simulink model "openWaterModel"  (R2020a)
settings: Solver=FixedStepAuto  StartTime=0.0  StopTime=inf  FixedStep=Ts  RelTol=1e-3  EnableMultiTasking=on
values from neighbouring files (symbols this model uses):
  ctrlMap =     [init_Kite.mat]
  Ts = 0.01    [init_Kite.mat]
undefined symbols (not defined in the file or in its folder): initializeBussesFromBlock, IO397, standard
libraries: xpcutilitieslib x172, hdlsllib x100, simulink x36, dspsigops x13, slrtlib x4, xpcseriallib x3, speedgoatlib_fpga_analog_io x2, xpcrtudplib x2, speedgoatlib_fpga_dio x1, speedgoatlib_fpga_quadrature x1, speedgoatlib_IO581 x1, speedgoatlib_fpga x1
(part 4 of 4)

== system openWaterModel/Sensor Processing/IMU Processing/Kite Measurements /binary2double3 ==
  In1 : Inport
  In2 : Inport  Port=2
  In3 : Inport  Port=3
  In4 : Inport  Port=4
  Bit Packing {,1..4} (5 alike) : xpcutilitieslib/Bit Packing 
      settings: SourceProductBaseCode=XP
  Bit Shift1 : hdlsllib/Logic and Bit Operations/Bit Shift  mode=Shift Left Logical  N=16
  Bit Shift2 : hdlsllib/Logic and Bit Operations/Bit Shift  mode=Shift Left Logical  N=24
  Bit Shift3 : hdlsllib/Logic and Bit Operations/Bit Shift  mode=Shift Left Logical  N=8
  Bitwise Operator : simulink/Logic and Bit Operations/Bitwise Operator  logicop=OR  UseBitMask=off  NumInputPorts=4  BitMask=bin2dec('00000000')  BitMaskRealWorld=Stored Integer
  Cast To Double1 : DataTypeConversion  OutDataTypeStr=double
  Display{3,5..7,10..14} (9 alike) : Display
      settings: Format=hex (Stored Integer)
  Double : Outport
  wires:
  Bit Shift1/1 -> Bitwise Operator/2, Display10/1
  Bitwise Operator/1 -> Display14/1, "Bit Packing "/1
  Bit Packing 1/1 -> Bit Shift2/1
  Bit Packing 4/1 -> Bitwise Operator/4, Display13/1
  In1/1 -> Bit Packing 1/1, Display3/1
  In3/1 -> Bit Packing 3/1, Display6/1
  Bit Shift2/1 -> Bitwise Operator/1, Display11/1
  Bit Packing 2/1 -> Bit Shift1/1
  "Bit Packing "/1 -> Cast To Double1/1
  Bit Shift3/1 -> Bitwise Operator/3, Display12/1
  Bit Packing 3/1 -> Bit Shift3/1
  In2/1 -> Bit Packing 2/1, Display5/1
  In4/1 -> Bit Packing 4/1, Display7/1
  Cast To Double1/1 -> Double/1

== system openWaterModel/Sensor Processing/IMU Processing/Kite Measurements /binary2double4 ==
  In1 : Inport
  In2 : Inport  Port=2
  In3 : Inport  Port=3
  In4 : Inport  Port=4
  Bit Packing {,1..4} (5 alike) : xpcutilitieslib/Bit Packing 
      settings: SourceProductBaseCode=XP
  Bit Shift1 : hdlsllib/Logic and Bit Operations/Bit Shift  mode=Shift Left Logical  N=16
  Bit Shift2 : hdlsllib/Logic and Bit Operations/Bit Shift  mode=Shift Left Logical  N=24
  Bit Shift3 : hdlsllib/Logic and Bit Operations/Bit Shift  mode=Shift Left Logical  N=8
  Bitwise Operator : simulink/Logic and Bit Operations/Bitwise Operator  logicop=OR  UseBitMask=off  NumInputPorts=4  BitMask=bin2dec('00000000')  BitMaskRealWorld=Stored Integer
  Cast To Double1 : DataTypeConversion  OutDataTypeStr=double
  Display{3,5..7,10..14} (9 alike) : Display
      settings: Format=hex (Stored Integer)
  Double : Outport
  wires:
  Bit Shift1/1 -> Bitwise Operator/2, Display10/1
  Bitwise Operator/1 -> Display14/1, "Bit Packing "/1
  Bit Packing 1/1 -> Bit Shift2/1
  Bit Packing 4/1 -> Bitwise Operator/4, Display13/1
  In1/1 -> Bit Packing 1/1, Display3/1
  In3/1 -> Bit Packing 3/1, Display6/1
  Bit Shift2/1 -> Bitwise Operator/1, Display11/1
  Bit Packing 2/1 -> Bit Shift1/1
  "Bit Packing "/1 -> Cast To Double1/1
  Bit Shift3/1 -> Bitwise Operator/3, Display12/1
  Bit Packing 3/1 -> Bit Shift3/1
  In2/1 -> Bit Packing 2/1, Display5/1
  In4/1 -> Bit Packing 4/1, Display7/1
  Cast To Double1/1 -> Double/1

== system openWaterModel/Sensor Processing/IMU Processing/Kite Measurements /binary2double5 ==
  In1 : Inport
  In2 : Inport  Port=2
  In3 : Inport  Port=3
  In4 : Inport  Port=4
  Bit Packing {,1..4} (5 alike) : xpcutilitieslib/Bit Packing 
      settings: SourceProductBaseCode=XP
  Bit Shift1 : hdlsllib/Logic and Bit Operations/Bit Shift  mode=Shift Left Logical  N=16
  Bit Shift2 : hdlsllib/Logic and Bit Operations/Bit Shift  mode=Shift Left Logical  N=24
  Bit Shift3 : hdlsllib/Logic and Bit Operations/Bit Shift  mode=Shift Left Logical  N=8
  Bitwise Operator : simulink/Logic and Bit Operations/Bitwise Operator  logicop=OR  UseBitMask=off  NumInputPorts=4  BitMask=bin2dec('00000000')  BitMaskRealWorld=Stored Integer
  Cast To Double1 : DataTypeConversion  OutDataTypeStr=double
  Display{3,5..7,10..14} (9 alike) : Display
      settings: Format=hex (Stored Integer)
  Double : Outport
  wires:
  Bit Shift1/1 -> Bitwise Operator/2, Display10/1
  Bitwise Operator/1 -> Display14/1, "Bit Packing "/1
  Bit Packing 1/1 -> Bit Shift2/1
  Bit Packing 4/1 -> Bitwise Operator/4, Display13/1
  In1/1 -> Bit Packing 1/1, Display3/1
  In3/1 -> Bit Packing 3/1, Display6/1
  Bit Shift2/1 -> Bitwise Operator/1, Display11/1
  Bit Packing 2/1 -> Bit Shift1/1
  "Bit Packing "/1 -> Cast To Double1/1
  Bit Shift3/1 -> Bitwise Operator/3, Display12/1
  Bit Packing 3/1 -> Bit Shift3/1
  In2/1 -> Bit Packing 2/1, Display5/1
  In4/1 -> Bit Packing 4/1, Display7/1
  Cast To Double1/1 -> Double/1

== system openWaterModel/Sensor Processing/IMU Processing/Kite Measurements /binary2double6 ==
  In1 : Inport
  In2 : Inport  Port=2
  In3 : Inport  Port=3
  In4 : Inport  Port=4
  Bit Packing {,1..4} (5 alike) : xpcutilitieslib/Bit Packing 
      settings: SourceProductBaseCode=XP
  Bit Shift1 : hdlsllib/Logic and Bit Operations/Bit Shift  mode=Shift Left Logical  N=16
  Bit Shift2 : hdlsllib/Logic and Bit Operations/Bit Shift  mode=Shift Left Logical  N=24
  Bit Shift3 : hdlsllib/Logic and Bit Operations/Bit Shift  mode=Shift Left Logical  N=8
  Bitwise Operator : simulink/Logic and Bit Operations/Bitwise Operator  logicop=OR  UseBitMask=off  NumInputPorts=4  BitMask=bin2dec('00000000')  BitMaskRealWorld=Stored Integer
  Cast To Double1 : DataTypeConversion  OutDataTypeStr=double
  Display{3,5..7,10..14} (9 alike) : Display
      settings: Format=hex (Stored Integer)
  Double : Outport
  wires:
  Bit Shift1/1 -> Bitwise Operator/2, Display10/1
  Bitwise Operator/1 -> Display14/1, "Bit Packing "/1
  Bit Packing 1/1 -> Bit Shift2/1
  Bit Packing 4/1 -> Bitwise Operator/4, Display13/1
  In1/1 -> Bit Packing 1/1, Display3/1
  In3/1 -> Bit Packing 3/1, Display6/1
  Bit Shift2/1 -> Bitwise Operator/1, Display11/1
  Bit Packing 2/1 -> Bit Shift1/1
  "Bit Packing "/1 -> Cast To Double1/1
  Bit Shift3/1 -> Bitwise Operator/3, Display12/1
  Bit Packing 3/1 -> Bit Shift3/1
  In2/1 -> Bit Packing 2/1, Display5/1
  In4/1 -> Bit Packing 4/1, Display7/1
  Cast To Double1/1 -> Double/1

== system openWaterModel/Sensor Processing/IMU Processing/Kite Measurements /binary2double7 ==
  In1 : Inport
  In2 : Inport  Port=2
  In3 : Inport  Port=3
  In4 : Inport  Port=4
  Bit Packing {,1..4} (5 alike) : xpcutilitieslib/Bit Packing 
      settings: SourceProductBaseCode=XP
  Bit Shift1 : hdlsllib/Logic and Bit Operations/Bit Shift  mode=Shift Left Logical  N=16
  Bit Shift2 : hdlsllib/Logic and Bit Operations/Bit Shift  mode=Shift Left Logical  N=24
  Bit Shift3 : hdlsllib/Logic and Bit Operations/Bit Shift  mode=Shift Left Logical  N=8
  Bitwise Operator : simulink/Logic and Bit Operations/Bitwise Operator  logicop=OR  UseBitMask=off  NumInputPorts=4  BitMask=bin2dec('00000000')  BitMaskRealWorld=Stored Integer
  Cast To Double1 : DataTypeConversion  OutDataTypeStr=double
  Display{3,5..7,10..14} (9 alike) : Display
      settings: Format=hex (Stored Integer)
  Double : Outport
  wires:
  Cast To Double1/1 -> Double/1
  In4/1 -> Display7/1, Bit Packing 4/1
  In2/1 -> Display5/1, Bit Packing 2/1
  Bit Packing 3/1 -> Bit Shift3/1
  Bit Shift3/1 -> Display12/1, Bitwise Operator/3
  "Bit Packing "/1 -> Cast To Double1/1
  Bit Packing 2/1 -> Bit Shift1/1
  Bit Shift2/1 -> Display11/1, Bitwise Operator/1
  In3/1 -> Display6/1, Bit Packing 3/1
  In1/1 -> Display3/1, Bit Packing 1/1
  Bit Packing 4/1 -> Display13/1, Bitwise Operator/4
  Bit Packing 1/1 -> Bit Shift2/1
  Bitwise Operator/1 -> "Bit Packing "/1, Display14/1
  Bit Shift1/1 -> Display10/1, Bitwise Operator/2

== system openWaterModel/Sensor Processing/IMU Processing/Kite Measurements /binary2double8 ==
  In1 : Inport
  In2 : Inport  Port=2
  In3 : Inport  Port=3
  In4 : Inport  Port=4
  Bit Packing {,1..4} (5 alike) : xpcutilitieslib/Bit Packing 
      settings: SourceProductBaseCode=XP
  Bit Shift1 : hdlsllib/Logic and Bit Operations/Bit Shift  mode=Shift Left Logical  N=16
  Bit Shift2 : hdlsllib/Logic and Bit Operations/Bit Shift  mode=Shift Left Logical  N=24
  Bit Shift3 : hdlsllib/Logic and Bit Operations/Bit Shift  mode=Shift Left Logical  N=8
  Bitwise Operator : simulink/Logic and Bit Operations/Bitwise Operator  logicop=OR  UseBitMask=off  NumInputPorts=4  BitMask=bin2dec('00000000')  BitMaskRealWorld=Stored Integer
  Cast To Double1 : DataTypeConversion  OutDataTypeStr=double
  Display{3,5..7,10..14} (9 alike) : Display
      settings: Format=hex (Stored Integer)
  Double : Outport
  wires:
  Bit Shift1/1 -> Bitwise Operator/2, Display10/1
  Bitwise Operator/1 -> Display14/1, "Bit Packing "/1
  Bit Packing 1/1 -> Bit Shift2/1
  Bit Packing 4/1 -> Bitwise Operator/4, Display13/1
  In1/1 -> Bit Packing 1/1, Display3/1
  In3/1 -> Bit Packing 3/1, Display6/1
  Bit Shift2/1 -> Bitwise Operator/1, Display11/1
  Bit Packing 2/1 -> Bit Shift1/1
  "Bit Packing "/1 -> Cast To Double1/1
  Bit Shift3/1 -> Bitwise Operator/3, Display12/1
  Bit Packing 3/1 -> Bit Shift3/1
  In2/1 -> Bit Packing 2/1, Display5/1
  In4/1 -> Bit Packing 4/1, Display7/1
  Cast To Double1/1 -> Double/1

== system openWaterModel/Sensor Processing/IMU Processing/Kite Measurements /binary2double9 ==
  In1 : Inport
  In2 : Inport  Port=2
  In3 : Inport  Port=3
  In4 : Inport  Port=4
  Bit Packing {,1..4} (5 alike) : xpcutilitieslib/Bit Packing 
      settings: SourceProductBaseCode=XP
  Bit Shift1 : hdlsllib/Logic and Bit Operations/Bit Shift  mode=Shift Left Logical  N=16
  Bit Shift2 : hdlsllib/Logic and Bit Operations/Bit Shift  mode=Shift Left Logical  N=24
  Bit Shift3 : hdlsllib/Logic and Bit Operations/Bit Shift  mode=Shift Left Logical  N=8
  Bitwise Operator : simulink/Logic and Bit Operations/Bitwise Operator  logicop=OR  UseBitMask=off  NumInputPorts=4  BitMask=bin2dec('00000000')  BitMaskRealWorld=Stored Integer
  Cast To Double1 : DataTypeConversion  OutDataTypeStr=double
  Display{3,5..7,10..14} (9 alike) : Display
      settings: Format=hex (Stored Integer)
  Double : Outport
  wires:
  Cast To Double1/1 -> Double/1
  In4/1 -> Display7/1, Bit Packing 4/1
  In2/1 -> Display5/1, Bit Packing 2/1
  Bit Packing 3/1 -> Bit Shift3/1
  Bit Shift3/1 -> Display12/1, Bitwise Operator/3
  "Bit Packing "/1 -> Cast To Double1/1
  Bit Packing 2/1 -> Bit Shift1/1
  Bit Shift2/1 -> Display11/1, Bitwise Operator/1
  In3/1 -> Display6/1, Bit Packing 3/1
  In1/1 -> Display3/1, Bit Packing 1/1
  Bit Packing 4/1 -> Display13/1, Bitwise Operator/4
  Bit Packing 1/1 -> Bit Shift2/1
  Bitwise Operator/1 -> "Bit Packing "/1, Display14/1
  Bit Shift1/1 -> Display10/1, Bitwise Operator/2

== system openWaterModel/Sensor Processing/IMU Processing/Kite Measurements /Serial Data Recieve/Enabled Subsystem ==
  Double : Inport
  Enable : EnablePort
  Out1 : Outport
  wires:
  Double/1 -> Out1/1

== system openWaterModel/Sensor Processing/IMU Processing/Kite Measurements /Serial Data Recieve/Enabled Subsystem1 ==
  Double : Inport
  Enable : EnablePort
  Out1 : Outport
  wires:
  Double/1 -> Out1/1

== system openWaterModel/Sensor Processing/IMU Processing/Kite Measurements /Serial Data Recieve/Enabled Subsystem2 ==
  Double : Inport
  Enable : EnablePort
  Out1 : Outport
  wires:
  Double/1 -> Out1/1

== system openWaterModel/Sensor Processing/IMU Processing/Kite Measurements /Serial Data Recieve/Enabled Subsystem3 ==
  Double : Inport
  Enable : EnablePort
  Out1 : Outport
  wires:
  Double/1 -> Out1/1

== system openWaterModel/Sensor Processing/IMU Processing/Kite Measurements /Serial Data Recieve/Enabled Subsystem4 ==
  Double : Inport
  Enable : EnablePort
  Out1 : Outport
  wires:
  Double/1 -> Out1/1

== system openWaterModel/Sensor Processing/IMU Processing/Kite Measurements /Serial Data Recieve/Enabled Subsystem5 ==
  Double : Inport
  Enable : EnablePort
  Out1 : Outport
  wires:
  Double/1 -> Out1/1

== system openWaterModel/Sensor Processing/IMU Processing/Kite Measurements /Serial Data Recieve/Enabled Subsystem6 ==
  Double : Inport
  Enable : EnablePort
  Out1 : Outport
  wires:
  Double/1 -> Out1/1

== system openWaterModel/Sensor Processing/IMU Processing/Kite Measurements /Serial Data Recieve/Enabled Subsystem7 ==
  Double : Inport
  Enable : EnablePort
  Out1 : Outport
  wires:
  Double/1 -> Out1/1

== system openWaterModel/Sensor Processing/IMU Processing/Kite Measurements /Serial Data Recieve/Enabled Subsystem8 ==
  Double : Inport
  Enable : EnablePort
  Out1 : Outport
  wires:
  Double/1 -> Out1/1

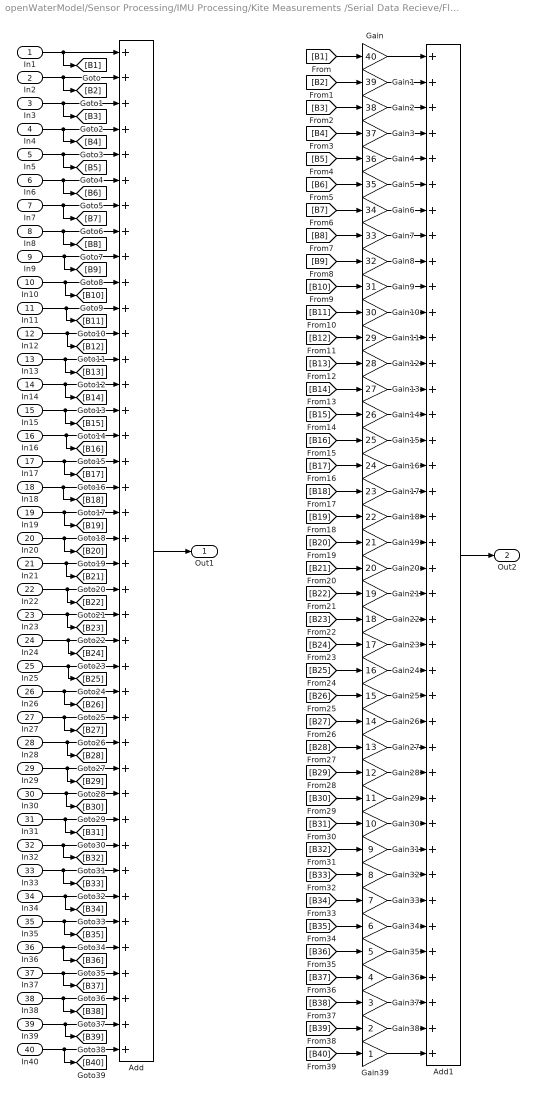
== system openWaterModel/Sensor Processing/IMU Processing/Kite Measurements /Serial Data Recieve/Fletcher16 Checksum ==
  In1 : Inport
  In2 : Inport  Port=2
  In3 : Inport  Port=3
  In4 : Inport  Port=4
  In5 : Inport  Port=5
  In6 : Inport  Port=6
  In7 : Inport  Port=7
  In8 : Inport  Port=8
  In9 : Inport  Port=9
  In10 : Inport  Port=10
  In11 : Inport  Port=11
  In12 : Inport  Port=12
  In13 : Inport  Port=13
  In14 : Inport  Port=14
  In15 : Inport  Port=15
  In16 : Inport  Port=16
  In17 : Inport  Port=17
  In18 : Inport  Port=18
  In19 : Inport  Port=19
  In20 : Inport  Port=20
  In21 : Inport  Port=21
  In22 : Inport  Port=22
  In23 : Inport  Port=23
  In24 : Inport  Port=24
  In25 : Inport  Port=25
  In26 : Inport  Port=26
  In27 : Inport  Port=27
  In28 : Inport  Port=28
  In29 : Inport  Port=29
  In30 : Inport  Port=30
  In31 : Inport  Port=31
  In32 : Inport  Port=32
  In33 : Inport  Port=33
  In34 : Inport  Port=34
  In35 : Inport  Port=35
  In36 : Inport  Port=36
  In37 : Inport  Port=37
  In38 : Inport  Port=38
  In39 : Inport  Port=39
  In40 : Inport  Port=40
  Add : Sum  Inputs=++++++++++++++++++++++++++++++++++++++++
  Add1 : Sum  Inputs=++++++++++++++++++++++++++++++++++++++++
  Gain : Gain  Gain=40  OutDataTypeStr=uint8
  Gain1 : Gain  Gain=39  OutDataTypeStr=uint8
  Gain10 : Gain  Gain=30  OutDataTypeStr=uint8
  Gain11 : Gain  Gain=29  OutDataTypeStr=uint8
  Gain12 : Gain  Gain=28  OutDataTypeStr=uint8
  Gain13 : Gain  Gain=27  OutDataTypeStr=uint8
  Gain14 : Gain  Gain=26  OutDataTypeStr=uint8
  Gain15 : Gain  Gain=25  OutDataTypeStr=uint8
  Gain16 : Gain  Gain=24  OutDataTypeStr=uint8
  Gain17 : Gain  Gain=23  OutDataTypeStr=uint8
  Gain18 : Gain  Gain=22  OutDataTypeStr=uint8
  Gain19 : Gain  Gain=21  OutDataTypeStr=uint8
  Gain2 : Gain  Gain=38  OutDataTypeStr=uint8
  Gain20 : Gain  Gain=20  OutDataTypeStr=uint8
  Gain21 : Gain  Gain=19  OutDataTypeStr=uint8
  Gain22 : Gain  Gain=18  OutDataTypeStr=uint8
  Gain23 : Gain  Gain=17  OutDataTypeStr=uint8
  Gain24 : Gain  Gain=16  OutDataTypeStr=uint8
  Gain25 : Gain  Gain=15  OutDataTypeStr=uint8
  Gain26 : Gain  Gain=14  OutDataTypeStr=uint8
  Gain27 : Gain  Gain=13  OutDataTypeStr=uint8
  Gain28 : Gain  Gain=12  OutDataTypeStr=uint8
  Gain29 : Gain  Gain=11  OutDataTypeStr=uint8
  Gain3 : Gain  Gain=37  OutDataTypeStr=uint8
  Gain30 : Gain  Gain=10  OutDataTypeStr=uint8
  Gain31 : Gain  Gain=9  OutDataTypeStr=uint8
  Gain32 : Gain  Gain=8  OutDataTypeStr=uint8
  Gain33 : Gain  Gain=7  OutDataTypeStr=uint8
  Gain34 : Gain  Gain=6  OutDataTypeStr=uint8
  Gain35 : Gain  Gain=5  OutDataTypeStr=uint8
  Gain36 : Gain  Gain=4  OutDataTypeStr=uint8
  Gain37 : Gain  Gain=3  OutDataTypeStr=uint8
  Gain38 : Gain  Gain=2  OutDataTypeStr=uint8
  Gain39 : Gain  OutDataTypeStr=uint8
  Gain4 : Gain  Gain=36  OutDataTypeStr=uint8
  Gain5 : Gain  Gain=35  OutDataTypeStr=uint8
  Gain6 : Gain  Gain=34  OutDataTypeStr=uint8
  Gain7 : Gain  Gain=33  OutDataTypeStr=uint8
  Gain8 : Gain  Gain=32  OutDataTypeStr=uint8
  Gain9 : Gain  Gain=31  OutDataTypeStr=uint8
  Out1 : Outport
  Out2 : Outport  Port=2
  wires:
  In3/1 -> [B3], Add/3
  [B4] -> Gain3/1
  In2/1 -> [B2], Add/2
  [B1] -> Gain/1
  Add1/1 -> Out2/1
  In4/1 -> [B4], Add/4
  [B3] -> Gain2/1
  In6/1 -> [B6], Add/6
  In5/1 -> [B5], Add/5
  [B2] -> Gain1/1
  [B5] -> Gain4/1
  In1/1 -> Add/1, [B1]
  Add/1 -> Out1/1
  In7/1 -> [B7], Add/7
  In8/1 -> [B8], Add/8
  In9/1 -> [B9], Add/9
  In10/1 -> [B10], Add/10
  In11/1 -> [B11], Add/11
  In12/1 -> [B12], Add/12
  In13/1 -> [B13], Add/13
  In14/1 -> [B14], Add/14
  In15/1 -> [B15], Add/15
  In16/1 -> [B16], Add/16
  In17/1 -> [B17], Add/17
  In18/1 -> [B18], Add/18
  In19/1 -> [B19], Add/19
  In20/1 -> [B20], Add/20
  In21/1 -> [B21], Add/21
  In22/1 -> [B22], Add/22
  In23/1 -> [B23], Add/23
  In24/1 -> [B24], Add/24
  In25/1 -> [B25], Add/25
  In26/1 -> [B26], Add/26
  In27/1 -> [B27], Add/27
  In28/1 -> [B28], Add/28
  In29/1 -> [B29], Add/29
  In30/1 -> [B30], Add/30
  In31/1 -> [B31], Add/31
  In32/1 -> [B32], Add/32
  In33/1 -> [B33], Add/33
  In34/1 -> [B34], Add/34
  In35/1 -> [B35], Add/35
  In36/1 -> [B36], Add/36
  In37/1 -> [B37], Add/37
  In38/1 -> [B38], Add/38
  In39/1 -> [B39], Add/39
  In40/1 -> [B40], Add/40
  Gain/1 -> Add1/1
  Gain1/1 -> Add1/2
  Gain2/1 -> Add1/3
  Gain3/1 -> Add1/4
  Gain4/1 -> Add1/5
  [B6] -> Gain5/1
  Gain5/1 -> Add1/6
  [B7] -> Gain6/1
  Gain6/1 -> Add1/7
  Gain7/1 -> Add1/8
  [B8] -> Gain7/1
  [B9] -> Gain8/1
  Gain8/1 -> Add1/9
  Gain9/1 -> Add1/10
  [B10] -> Gain9/1
  [B11] -> Gain10/1
  Gain10/1 -> Add1/11
  [B12] -> Gain11/1
  [B13] -> Gain12/1
  [B14] -> Gain13/1
  Gain13/1 -> Add1/14
  [B15] -> Gain14/1
  Gain14/1 -> Add1/15
  [B16] -> Gain15/1
  Gain15/1 -> Add1/16
  [B17] -> Gain16/1
  Gain16/1 -> Add1/17
  [B18] -> Gain17/1
  Gain17/1 -> Add1/18
  [B19] -> Gain18/1
  Gain18/1 -> Add1/19
  [B20] -> Gain19/1
  Gain19/1 -> Add1/20
  [B21] -> Gain20/1
  Gain20/1 -> Add1/21
  [B22] -> Gain21/1
  Gain21/1 -> Add1/22
  [B23] -> Gain22/1
  Gain22/1 -> Add1/23
  [B24] -> Gain23/1
  Gain23/1 -> Add1/24
  [B25] -> Gain24/1
  Gain24/1 -> Add1/25
  [B26] -> Gain25/1
  Gain25/1 -> Add1/26
  [B27] -> Gain26/1
  Gain26/1 -> Add1/27
  [B28] -> Gain27/1
  Gain27/1 -> Add1/28
  [B29] -> Gain28/1
  Gain28/1 -> Add1/29
  [B30] -> Gain29/1
  Gain29/1 -> Add1/30
  [B31] -> Gain30/1
  Gain30/1 -> Add1/31
  [B32] -> Gain31/1
  Gain31/1 -> Add1/32
  [B33] -> Gain32/1
  Gain32/1 -> Add1/33
  [B34] -> Gain33/1
  Gain33/1 -> Add1/34
  [B35] -> Gain34/1
  Gain34/1 -> Add1/35
  [B36] -> Gain35/1
  Gain35/1 -> Add1/36
  [B37] -> Gain36/1
  Gain36/1 -> Add1/37
  [B38] -> Gain37/1
  Gain37/1 -> Add1/38
  [B39] -> Gain38/1
  Gain38/1 -> Add1/39
  [B40] -> Gain39/1
  Gain39/1 -> Add1/40
  Gain11/1 -> Add1/12
  Gain12/1 -> Add1/13

== system openWaterModel/Sensor Processing/IMU Processing/Kite Measurements /Serial Data Recieve/binary2double ==
  In1 : Inport
  In2 : Inport  Port=2
  In3 : Inport  Port=3
  In4 : Inport  Port=4
  Bit Packing {,1..4} (5 alike) : xpcutilitieslib/Bit Packing 
      settings: SourceProductBaseCode=XP
  Bit Shift1 : hdlsllib/Logic and Bit Operations/Bit Shift  mode=Shift Left Logical  N=16
  Bit Shift2 : hdlsllib/Logic and Bit Operations/Bit Shift  mode=Shift Left Logical  N=24
  Bit Shift3 : hdlsllib/Logic and Bit Operations/Bit Shift  mode=Shift Left Logical  N=8
  Bitwise Operator : simulink/Logic and Bit Operations/Bitwise Operator  logicop=OR  UseBitMask=off  NumInputPorts=4  BitMask=bin2dec('00000000')  BitMaskRealWorld=Stored Integer
  Cast To Double1 : DataTypeConversion  OutDataTypeStr=double
  Display{3,5..7,10..14} (9 alike) : Display
      settings: Format=hex (Stored Integer)
  Double : Outport
  wires:
  Bit Shift1/1 -> Bitwise Operator/2, Display10/1
  Bitwise Operator/1 -> Display14/1, "Bit Packing "/1
  Bit Packing 1/1 -> Bit Shift2/1
  Bit Packing 4/1 -> Bitwise Operator/4, Display13/1
  In1/1 -> Bit Packing 1/1, Display3/1
  In3/1 -> Bit Packing 3/1, Display6/1
  Bit Shift2/1 -> Bitwise Operator/1, Display11/1
  Bit Packing 2/1 -> Bit Shift1/1
  "Bit Packing "/1 -> Cast To Double1/1
  Bit Shift3/1 -> Bitwise Operator/3, Display12/1
  Bit Packing 3/1 -> Bit Shift3/1
  In2/1 -> Bit Packing 2/1, Display5/1
  In4/1 -> Bit Packing 4/1, Display7/1
  Cast To Double1/1 -> Double/1

== system openWaterModel/Sensor Processing/IMU Processing/Kite Measurements /Serial Data Recieve/binary2double1 ==
  In1 : Inport
  In2 : Inport  Port=2
  In3 : Inport  Port=3
  In4 : Inport  Port=4
  Bit Packing {,1..4} (5 alike) : xpcutilitieslib/Bit Packing 
      settings: SourceProductBaseCode=XP
  Bit Shift1 : hdlsllib/Logic and Bit Operations/Bit Shift  mode=Shift Left Logical  N=16
  Bit Shift2 : hdlsllib/Logic and Bit Operations/Bit Shift  mode=Shift Left Logical  N=24
  Bit Shift3 : hdlsllib/Logic and Bit Operations/Bit Shift  mode=Shift Left Logical  N=8
  Bitwise Operator : simulink/Logic and Bit Operations/Bitwise Operator  logicop=OR  UseBitMask=off  NumInputPorts=4  BitMask=bin2dec('00000000')  BitMaskRealWorld=Stored Integer
  Cast To Double1 : DataTypeConversion  OutDataTypeStr=double
  Display{3,5..7,10..14} (9 alike) : Display
      settings: Format=hex (Stored Integer)
  Double : Outport
  wires:
  Bit Shift1/1 -> Bitwise Operator/2, Display10/1
  Bitwise Operator/1 -> Display14/1, "Bit Packing "/1
  Bit Packing 1/1 -> Bit Shift2/1
  Bit Packing 4/1 -> Bitwise Operator/4, Display13/1
  In1/1 -> Bit Packing 1/1, Display3/1
  In3/1 -> Bit Packing 3/1, Display6/1
  Bit Shift2/1 -> Bitwise Operator/1, Display11/1
  Bit Packing 2/1 -> Bit Shift1/1
  "Bit Packing "/1 -> Cast To Double1/1
  Bit Shift3/1 -> Bitwise Operator/3, Display12/1
  Bit Packing 3/1 -> Bit Shift3/1
  In2/1 -> Bit Packing 2/1, Display5/1
  In4/1 -> Bit Packing 4/1, Display7/1
  Cast To Double1/1 -> Double/1

== system openWaterModel/Sensor Processing/IMU Processing/Kite Measurements /Serial Data Recieve/binary2double2 ==
  In1 : Inport
  In2 : Inport  Port=2
  In3 : Inport  Port=3
  In4 : Inport  Port=4
  Bit Packing {,1..4} (5 alike) : xpcutilitieslib/Bit Packing 
      settings: SourceProductBaseCode=XP
  Bit Shift1 : hdlsllib/Logic and Bit Operations/Bit Shift  mode=Shift Left Logical  N=16
  Bit Shift2 : hdlsllib/Logic and Bit Operations/Bit Shift  mode=Shift Left Logical  N=24
  Bit Shift3 : hdlsllib/Logic and Bit Operations/Bit Shift  mode=Shift Left Logical  N=8
  Bitwise Operator : simulink/Logic and Bit Operations/Bitwise Operator  logicop=OR  UseBitMask=off  NumInputPorts=4  BitMask=bin2dec('00000000')  BitMaskRealWorld=Stored Integer
  Cast To Double1 : DataTypeConversion  OutDataTypeStr=double
  Display{3,5..7,10..14} (9 alike) : Display
      settings: Format=hex (Stored Integer)
  Double : Outport
  wires:
  Bit Shift1/1 -> Bitwise Operator/2, Display10/1
  Bitwise Operator/1 -> Display14/1, "Bit Packing "/1
  Bit Packing 1/1 -> Bit Shift2/1
  Bit Packing 4/1 -> Bitwise Operator/4, Display13/1
  In1/1 -> Bit Packing 1/1, Display3/1
  In3/1 -> Bit Packing 3/1, Display6/1
  Bit Shift2/1 -> Bitwise Operator/1, Display11/1
  Bit Packing 2/1 -> Bit Shift1/1
  "Bit Packing "/1 -> Cast To Double1/1
  Bit Shift3/1 -> Bitwise Operator/3, Display12/1
  Bit Packing 3/1 -> Bit Shift3/1
  In2/1 -> Bit Packing 2/1, Display5/1
  In4/1 -> Bit Packing 4/1, Display7/1
  Cast To Double1/1 -> Double/1

== system openWaterModel/Sensor Processing/IMU Processing/Kite Measurements /Serial Data Recieve/binary2double3 ==
  In1 : Inport
  In2 : Inport  Port=2
  In3 : Inport  Port=3
  In4 : Inport  Port=4
  Bit Packing {,1..4} (5 alike) : xpcutilitieslib/Bit Packing 
      settings: SourceProductBaseCode=XP
  Bit Shift1 : hdlsllib/Logic and Bit Operations/Bit Shift  mode=Shift Left Logical  N=16
  Bit Shift2 : hdlsllib/Logic and Bit Operations/Bit Shift  mode=Shift Left Logical  N=24
  Bit Shift3 : hdlsllib/Logic and Bit Operations/Bit Shift  mode=Shift Left Logical  N=8
  Bitwise Operator : simulink/Logic and Bit Operations/Bitwise Operator  logicop=OR  UseBitMask=off  NumInputPorts=4  BitMask=bin2dec('00000000')  BitMaskRealWorld=Stored Integer
  Cast To Double1 : DataTypeConversion  OutDataTypeStr=double
  Display{3,5..7,10..14} (9 alike) : Display
      settings: Format=hex (Stored Integer)
  Double : Outport
  wires:
  Bit Shift1/1 -> Bitwise Operator/2, Display10/1
  Bitwise Operator/1 -> Display14/1, "Bit Packing "/1
  Bit Packing 1/1 -> Bit Shift2/1
  Bit Packing 4/1 -> Bitwise Operator/4, Display13/1
  In1/1 -> Bit Packing 1/1, Display3/1
  In3/1 -> Bit Packing 3/1, Display6/1
  Bit Shift2/1 -> Bitwise Operator/1, Display11/1
  Bit Packing 2/1 -> Bit Shift1/1
  "Bit Packing "/1 -> Cast To Double1/1
  Bit Shift3/1 -> Bitwise Operator/3, Display12/1
  Bit Packing 3/1 -> Bit Shift3/1
  In2/1 -> Bit Packing 2/1, Display5/1
  In4/1 -> Bit Packing 4/1, Display7/1
  Cast To Double1/1 -> Double/1

== system openWaterModel/Sensor Processing/IMU Processing/Kite Measurements /Serial Data Recieve/binary2double4 ==
  In1 : Inport
  In2 : Inport  Port=2
  In3 : Inport  Port=3
  In4 : Inport  Port=4
  Bit Packing {,1..4} (5 alike) : xpcutilitieslib/Bit Packing 
      settings: SourceProductBaseCode=XP
  Bit Shift1 : hdlsllib/Logic and Bit Operations/Bit Shift  mode=Shift Left Logical  N=16
  Bit Shift2 : hdlsllib/Logic and Bit Operations/Bit Shift  mode=Shift Left Logical  N=24
  Bit Shift3 : hdlsllib/Logic and Bit Operations/Bit Shift  mode=Shift Left Logical  N=8
  Bitwise Operator : simulink/Logic and Bit Operations/Bitwise Operator  logicop=OR  UseBitMask=off  NumInputPorts=4  BitMask=bin2dec('00000000')  BitMaskRealWorld=Stored Integer
  Cast To Double1 : DataTypeConversion  OutDataTypeStr=double
  Display{3,5..7,10..14} (9 alike) : Display
      settings: Format=hex (Stored Integer)
  Double : Outport
  wires:
  Bit Shift1/1 -> Bitwise Operator/2, Display10/1
  Bitwise Operator/1 -> Display14/1, "Bit Packing "/1
  Bit Packing 1/1 -> Bit Shift2/1
  Bit Packing 4/1 -> Bitwise Operator/4, Display13/1
  In1/1 -> Bit Packing 1/1, Display3/1
  In3/1 -> Bit Packing 3/1, Display6/1
  Bit Shift2/1 -> Bitwise Operator/1, Display11/1
  Bit Packing 2/1 -> Bit Shift1/1
  "Bit Packing "/1 -> Cast To Double1/1
  Bit Shift3/1 -> Bitwise Operator/3, Display12/1
  Bit Packing 3/1 -> Bit Shift3/1
  In2/1 -> Bit Packing 2/1, Display5/1
  In4/1 -> Bit Packing 4/1, Display7/1
  Cast To Double1/1 -> Double/1

== system openWaterModel/Sensor Processing/IMU Processing/Kite Measurements /Serial Data Recieve/binary2double5 ==
  In1 : Inport
  In2 : Inport  Port=2
  In3 : Inport  Port=3
  In4 : Inport  Port=4
  Bit Packing {,1..4} (5 alike) : xpcutilitieslib/Bit Packing 
      settings: SourceProductBaseCode=XP
  Bit Shift1 : hdlsllib/Logic and Bit Operations/Bit Shift  mode=Shift Left Logical  N=16
  Bit Shift2 : hdlsllib/Logic and Bit Operations/Bit Shift  mode=Shift Left Logical  N=24
  Bit Shift3 : hdlsllib/Logic and Bit Operations/Bit Shift  mode=Shift Left Logical  N=8
  Bitwise Operator : simulink/Logic and Bit Operations/Bitwise Operator  logicop=OR  UseBitMask=off  NumInputPorts=4  BitMask=bin2dec('00000000')  BitMaskRealWorld=Stored Integer
  Cast To Double1 : DataTypeConversion  OutDataTypeStr=double
  Display{3,5..7,10..14} (9 alike) : Display
      settings: Format=hex (Stored Integer)
  Double : Outport
  wires:
  Bit Shift1/1 -> Bitwise Operator/2, Display10/1
  Bitwise Operator/1 -> Display14/1, "Bit Packing "/1
  Bit Packing 1/1 -> Bit Shift2/1
  Bit Packing 4/1 -> Bitwise Operator/4, Display13/1
  In1/1 -> Bit Packing 1/1, Display3/1
  In3/1 -> Bit Packing 3/1, Display6/1
  Bit Shift2/1 -> Bitwise Operator/1, Display11/1
  Bit Packing 2/1 -> Bit Shift1/1
  "Bit Packing "/1 -> Cast To Double1/1
  Bit Shift3/1 -> Bitwise Operator/3, Display12/1
  Bit Packing 3/1 -> Bit Shift3/1
  In2/1 -> Bit Packing 2/1, Display5/1
  In4/1 -> Bit Packing 4/1, Display7/1
  Cast To Double1/1 -> Double/1

== system openWaterModel/Sensor Processing/IMU Processing/Kite Measurements /Serial Data Recieve/binary2double6 ==
  In1 : Inport
  In2 : Inport  Port=2
  In3 : Inport  Port=3
  In4 : Inport  Port=4
  Bit Packing {,1..4} (5 alike) : xpcutilitieslib/Bit Packing 
      settings: SourceProductBaseCode=XP
  Bit Shift1 : hdlsllib/Logic and Bit Operations/Bit Shift  mode=Shift Left Logical  N=16
  Bit Shift2 : hdlsllib/Logic and Bit Operations/Bit Shift  mode=Shift Left Logical  N=24
  Bit Shift3 : hdlsllib/Logic and Bit Operations/Bit Shift  mode=Shift Left Logical  N=8
  Bitwise Operator : simulink/Logic and Bit Operations/Bitwise Operator  logicop=OR  UseBitMask=off  NumInputPorts=4  BitMask=bin2dec('00000000')  BitMaskRealWorld=Stored Integer
  Cast To Double1 : DataTypeConversion  OutDataTypeStr=double
  Display{3,5..7,10..14} (9 alike) : Display
      settings: Format=hex (Stored Integer)
  Double : Outport
  wires:
  Bit Shift1/1 -> Bitwise Operator/2, Display10/1
  Bitwise Operator/1 -> Display14/1, "Bit Packing "/1
  Bit Packing 1/1 -> Bit Shift2/1
  Bit Packing 4/1 -> Bitwise Operator/4, Display13/1
  In1/1 -> Bit Packing 1/1, Display3/1
  In3/1 -> Bit Packing 3/1, Display6/1
  Bit Shift2/1 -> Bitwise Operator/1, Display11/1
  Bit Packing 2/1 -> Bit Shift1/1
  "Bit Packing "/1 -> Cast To Double1/1
  Bit Shift3/1 -> Bitwise Operator/3, Display12/1
  Bit Packing 3/1 -> Bit Shift3/1
  In2/1 -> Bit Packing 2/1, Display5/1
  In4/1 -> Bit Packing 4/1, Display7/1
  Cast To Double1/1 -> Double/1

== system openWaterModel/Sensor Processing/IMU Processing/Kite Measurements /Serial Data Recieve/binary2double7 ==
  In1 : Inport
  In2 : Inport  Port=2
  In3 : Inport  Port=3
  In4 : Inport  Port=4
  Bit Packing {,1..4} (5 alike) : xpcutilitieslib/Bit Packing 
      settings: SourceProductBaseCode=XP
  Bit Shift1 : hdlsllib/Logic and Bit Operations/Bit Shift  mode=Shift Left Logical  N=16
  Bit Shift2 : hdlsllib/Logic and Bit Operations/Bit Shift  mode=Shift Left Logical  N=24
  Bit Shift3 : hdlsllib/Logic and Bit Operations/Bit Shift  mode=Shift Left Logical  N=8
  Bitwise Operator : simulink/Logic and Bit Operations/Bitwise Operator  logicop=OR  UseBitMask=off  NumInputPorts=4  BitMask=bin2dec('00000000')  BitMaskRealWorld=Stored Integer
  Cast To Double1 : DataTypeConversion  OutDataTypeStr=double
  Display{3,5..7,10..14} (9 alike) : Display
      settings: Format=hex (Stored Integer)
  Double : Outport
  wires:
  Cast To Double1/1 -> Double/1
  In4/1 -> Display7/1, Bit Packing 4/1
  In2/1 -> Display5/1, Bit Packing 2/1
  Bit Packing 3/1 -> Bit Shift3/1
  Bit Shift3/1 -> Display12/1, Bitwise Operator/3
  "Bit Packing "/1 -> Cast To Double1/1
  Bit Packing 2/1 -> Bit Shift1/1
  Bit Shift2/1 -> Display11/1, Bitwise Operator/1
  In3/1 -> Display6/1, Bit Packing 3/1
  In1/1 -> Display3/1, Bit Packing 1/1
  Bit Packing 4/1 -> Display13/1, Bitwise Operator/4
  Bit Packing 1/1 -> Bit Shift2/1
  Bitwise Operator/1 -> "Bit Packing "/1, Display14/1
  Bit Shift1/1 -> Display10/1, Bitwise Operator/2

== system openWaterModel/Sensor Processing/IMU Processing/Kite Measurements /Serial Data Recieve/binary2double8 ==
  In1 : Inport
  In2 : Inport  Port=2
  In3 : Inport  Port=3
  In4 : Inport  Port=4
  Bit Packing {,1..4} (5 alike) : xpcutilitieslib/Bit Packing 
      settings: SourceProductBaseCode=XP
  Bit Shift1 : hdlsllib/Logic and Bit Operations/Bit Shift  mode=Shift Left Logical  N=16
  Bit Shift2 : hdlsllib/Logic and Bit Operations/Bit Shift  mode=Shift Left Logical  N=24
  Bit Shift3 : hdlsllib/Logic and Bit Operations/Bit Shift  mode=Shift Left Logical  N=8
  Bitwise Operator : simulink/Logic and Bit Operations/Bitwise Operator  logicop=OR  UseBitMask=off  NumInputPorts=4  BitMask=bin2dec('00000000')  BitMaskRealWorld=Stored Integer
  Cast To Double1 : DataTypeConversion  OutDataTypeStr=double
  Display{3,5..7,10..14} (9 alike) : Display
      settings: Format=hex (Stored Integer)
  Double : Outport
  wires:
  Bit Shift1/1 -> Bitwise Operator/2, Display10/1
  Bitwise Operator/1 -> Display14/1, "Bit Packing "/1
  Bit Packing 1/1 -> Bit Shift2/1
  Bit Packing 4/1 -> Bitwise Operator/4, Display13/1
  In1/1 -> Bit Packing 1/1, Display3/1
  In3/1 -> Bit Packing 3/1, Display6/1
  Bit Shift2/1 -> Bitwise Operator/1, Display11/1
  Bit Packing 2/1 -> Bit Shift1/1
  "Bit Packing "/1 -> Cast To Double1/1
  Bit Shift3/1 -> Bitwise Operator/3, Display12/1
  Bit Packing 3/1 -> Bit Shift3/1
  In2/1 -> Bit Packing 2/1, Display5/1
  In4/1 -> Bit Packing 4/1, Display7/1
  Cast To Double1/1 -> Double/1

== matlab function openWaterModel/Euler setpoints /MATLAB Function4 ==
  data: u input; rollSP output; pitchSP output; yawSP output
function [rollSP,pitchSP, yawSP] = fcn(u)

rollSP = u(1);
pitchSP = u(2);
yawSP = u(3);

end

== matlab function openWaterModel/MATLAB Function4 ==
  data: triggType input; triggON output; clck input; timeTrigg input; speed input; speedTrigg input; pos input; posTrigg input; manualTrigg input
function triggON  = fcn(triggType, clck,timeTrigg,speed,speedTrigg,pos,posTrigg,manualTrigg)
%Control Trigger
% 1 = time, 2 = speed, 3 = position, 0 = manual
triggON=0;
if triggType == 1
    if clck > timeTrigg
        triggON = 1;
    end
elseif triggType ==2 
    if speed > speedTrigg
        triggON =1;
    end
elseif triggType ==3
    if pos > posTrigg
        triggON =1;
    end
elseif triggType ==0 && manualTrigg == 1
    triggON = 1;
end
    
    

end

== matlab function openWaterModel/MATLAB Function1 ==
  data: rollSP input; y output; pitchSP input; yawSP input
function y = fcn(rollSP, pitchSP,yawSP)

y = [rollSP pitchSP yawSP];


end

== matlab function openWaterModel/Sensor Processing/IMU Processing/Kite Measurements /MATLAB Function1 ==
  data: u input; y output
function y = fcn(u)
    if abs(u)>20
        y = 0;
    else
        y = u;
    end
end

== matlab function openWaterModel/Sensor Processing/LAS_Calculation/ifOutsideBounds ==
  data: u input; y output
function y = fcn(u)

if u > 180
    u = u - 360;
elseif u < -180
    u = u + 360;    
end

y = u;

== matlab function openWaterModel/Sensor Processing/IMU Processing/Kite Measurements /MATLAB Function2 ==
  data: u input; y output
function y = fcn(u)
    if abs(u)>20
        y = 0;
    else
        y = u;
    end
end

== matlab function openWaterModel/Sensor Processing/IMU Processing/Kite Measurements /Serial Data Recieve/MATLAB Function3 ==
  data: cSumInB1 input; checksumIsMatching output; cSumInB2 input; cSumCalcB1 input; cSumCalcB2 input
function checksumIsMatching = fcn(cSumInB1,cSumInB2,cSumCalcB1,cSumCalcB2)
    if cSumInB1 == cSumCalcB1 && cSumInB2 == cSumCalcB2
        checksumIsMatching = 1;
    else
        checksumIsMatching = 0;
    end
end

== matlab function openWaterModel/Euler setpoints /MATLAB Function1 ==
  data: tZcurr input; y output; tZeroAmp input
function y = fcn(tZcurr, tZeroAmp)

if tZcurr > tZeroAmp
    y = 0;
else
    y =1;
end

end

== matlab function openWaterModel/Sensor Processing/IMU Processing/Kite Measurements /MATLAB Function3 ==
  data: phi input; psi_dot output; theta input; q input; r input
function psi_dot = fcn(phi, theta, q, r)
% phi = roll angle; theta = pitch angle
% q = pitch rate; r = yaw rate
term1 = q*sin(phi)/cos(theta);
term2 = r*cos(phi)/cos(theta);

psi_dot = term1 + term2;
end

== matlab function openWaterModel/Sensor Processing/IMU Processing/Kite Measurements /MATLAB Function4 ==
  data: u input; y output
function y = fcn(u)
    if abs(u)>20
        y = 0;
    else
        y = u;
    end
end

== matlab function openWaterModel/Sensor Processing/IMU Processing/Kite Measurements /MATLAB Function5 ==
  data: u input; y output
function y = fcn(u)
    if abs(u)>20
        y = 0;
    else
        y = u;
    end
end

== matlab function openWaterModel/Sensor Processing/IMU Processing/Kite Measurements /MATLAB Function6 ==
  data: cSumInB1 input; checksumIsMatching output; cSumInB2 input; cSumCalcB1 input; cSumCalcB2 input
function checksumIsMatching = fcn(cSumInB1,cSumInB2,cSumCalcB1,cSumCalcB2)
    if cSumInB1 == cSumCalcB1 && cSumInB2 == cSumCalcB2
        checksumIsMatching = 1;
    else
        checksumIsMatching = 0;
    end
end

== matlab function openWaterModel/Sensor Processing/IMU Processing/Kite Measurements /MATLAB Function7 ==
  data: cSumInB1 input; checksumIsMatching output; cSumInB2 input; cSumCalcB1 input; cSumCalcB2 input
function checksumIsMatching = fcn(cSumInB1,cSumInB2,cSumCalcB1,cSumCalcB2)
    if cSumInB1 == cSumCalcB1 && cSumInB2 == cSumCalcB2
        checksumIsMatching = 1;
    else
        checksumIsMatching = 0;
    end
end

== matlab function openWaterModel/Sensor Processing/LAS_Calculation/LAS Measurement Corrections ==
  data: elev output; elev_encoder input; azi output; azi_encoder input
function [elev,azi] = fcn(elev_encoder, azi_encoder)

% Roller radius
rollRad = 0.0381;   % m

% Elevation joint, azimuth hub
elLink.a = 0.0229997;   % m
elLink.alpha = -pi/2;   % rad
elLink.d = 0;
elLink.theta = -elev_encoder; % Elevation encoder (change to pipe in data)

% Azimuth joint, boom
azLink.a = 0.49424;  % m
azLink.alpha = 0;
azLink.d = 0.0304;   % m
azLink.theta = azi_encoder; % Azimuth encoder (change to pipe in data)

% Elevation joint to end effector
Ael = jointTform(elLink);
Aaz = jointTform(azLink);
T = Ael*Aaz; % Transformation matrix

% Information above will be used in dynamics calculations
% --------------------------------------------------------------
% Information below is used for correcting tether angle
% Assume that the tether is tangent to the roller

endEffCart = T(1:3,4); % Enf effector Cartesian coordinates

% Roller center to end effector
hubCart = [-0.0717;-0.06785;0]; % Roller center to elevation joint
rc2ef = hubCart + endEffCart;

% Magnitude of roll center to end effector (2D)
rc2ef_Hyp = sqrt(rc2ef(1)^2 + rc2ef(2)^2);

% Elevation angle between end eff. to center and end eff. to surface
thetaOppHyp = asin(rollRad/rc2ef_Hyp);

% Elevation angle between end eff. to center and horizontal
thetaElevation = asin(-rc2ef(2)/rc2ef_Hyp);

% Angle from vertical to tether contact point on the roller
rollAng = thetaElevation-thetaOppHyp;

% Vector approximation from roller center to contact surface
% Map roller contact angle to elevation angle
rc2rsApprox = [cos(elLink.theta) -sin(elLink.theta) 0;
              sin(elLink.theta) cos(elLink.theta)   0;
              0                 0                   1]*[0;-rollRad;0];

% Vector from roller center to contact surface
% Using center-surface angle determined by trig
rc2rs = [cos(-rollAng) -sin(-rollAng) 0;
        sin(-rollAng)  cos(-rollAng)  0;
        0              0              1]*[0;-rollRad;0];

% Vector from contact surface to end effector (APPROXIMATION)
tetherVecApprox = rc2ef - rc2rsApprox;

% Vector from contact surface to end effector (FINAL)
tetherVec = rc2ef - rc2rs;

%% Block output

% Change block output spherical
    elev = asin(-tetherVecApprox(2)/norm(tetherVecApprox));
    azi = asin(-tetherVecApprox(3)/norm(tetherVecApprox)/cos(elev));

end

function A = jointTform(link)

% Transforms from the end effector to the base frame in the order: joint
% angle, then link offset, then link 

% INPUT %
% link.theta - joint angle (radians)
% link.d     - link offset
% link.a     - link length
% linkalpha - link twist (radians)

% OUTPUT %
% A - homogeneous transform matrix

At = [cos(link.theta) -sin(link.theta) 0 0;...
      sin(link.theta) cos(link.theta) 0 0;...
      0 0 1 0; 0 0 0 1];
  
Ad = [1 0 0 0; 0 1 0 0; 0 0 1 link.d; 0 0 0 1];

Aa = [1 0 0 link.a; 0 1 0 0; 0 0 1 0; 0 0 0 1];

Al = [1 0 0 0; 0 cos(link.alpha) -sin(link.alpha) 0;
      0 sin(link.alpha) cos(link.alpha) 0; 0 0 0 1];
  
A = At*Ad*Aa*Al;
end

== matlab function openWaterModel/Sensor Processing/IMU Processing/Kite Measurements /MATLAB Function8 ==
  data: cSumInB1 input; checksumIsMatching output; cSumInB2 input; cSumCalcB1 input; cSumCalcB2 input
function checksumIsMatching = fcn(cSumInB1,cSumInB2,cSumCalcB1,cSumCalcB2)
    if cSumInB1 == cSumCalcB1 && cSumInB2 == cSumCalcB2
        checksumIsMatching = 1;
    else
        checksumIsMatching = 0;
    end
end

== matlab function openWaterModel/Sensor Processing/LAS_Calculation/ifOutsideBounds1 ==
  data: u input; y output
function y = fcn(u)

if u > 180
    u = u - 360;
elseif u < -180
    u = u + 360;    
end

y = u;

== matlab function openWaterModel/Euler setpoints /MATLAB Function ==
  data: y output; t input
function y = fcn(t)
% ws = load('data_07_May_2021_13_02_14.mat');
speeddata;
y = t;
end

== matlab function openWaterModel/Sensor Processing/Subsystem1/Subsystem1/MATLAB Function ==
  data: el input; x1 output; az input; thrLength input; x2 output; x3 output
function [x1,x2,x3] = fcn(el,az,thrLength)
L = thrLength; 

x1 = L*cos(el)*cos(az); 
x2 = L*cos(el)*sin(az); 
x3 = L*sin(el);

== matlab function openWaterModel/MATLAB Function2 ==
  data: u input; y output
function y = fcn(u)
y = repmat(u,1,13);

== matlab function openWaterModel/Sensor Processing/IMU Processing/Kite Measurements /MATLAB Function ==
  data: phi input; psi_dot output; theta input; q input; r input
function psi_dot = fcn(phi, theta, q, r)
% phi = roll angle; theta = pitch angle
% q = pitch rate; r = yaw rate
term1 = q*sin(phi)/cos(theta);
term2 = r*cos(phi)/cos(theta);

psi_dot = term1 + term2;
end

== matlab function openWaterModel/Euler setpoints /RollSPTrigger ==
  data: trigg input; Const output; Sine output; Square output; SPType input
function [Const, Sine, Square] = fcn(trigg,SPType)
Const = 0;
Sine = 0;
Square = 0;

if SPType == 1
    if trigg == 1
        Const = 1;
    end
elseif SPType == 2
    if trigg ==1
        Sine = 1;
    end
elseif SPType ==3
    if trigg ==1
        Square = 1;
    end
end
end

== matlab function openWaterModel/Euler setpoints /YawSPTrigger ==
  data: trigg input; Const output; Sine output; Square output; SPType input
function [Const, Sine, Square] = fcn(trigg,SPType)
Const = 0;
Sine = 0;
Square = 0;

if SPType == 1
    if trigg == 1
        Const = 1;
    end
elseif SPType == 2
    if trigg ==1
        Sine = 1;
    end
elseif SPType ==3
    if trigg ==1
        Square = 1;
    end
end
end

== matlab function openWaterModel/Euler setpoints /PitchSPTrigger ==
  data: trigg input; Const output; Sine output; Square output; SPType input
function [Const, Sine, Square] = fcn(trigg,SPType)
Const = 0;
Sine = 0;
Square = 0;

if SPType == 1
    if trigg == 1
        Const = 1;
    end
elseif SPType == 2
    if trigg ==1
        Sine = 1;
    end
elseif SPType ==3
    if trigg ==1
        Square = 1;
    end
end
end
